simulink model "SVPWM"  (R2021a)
settings: Solver=FixedStepAuto  StartTime=0.0  StopTime=0.02  FixedStep=1e-7  RelTol=1e-3
values from neighbouring files (symbols this model uses):
  f_fund = 50    [run_sim.m]
  ma = 0.2    [run_sim.m]
  phaseA = 0    [run_sim.m]
  phi_carrier = 0    [run_sim.m]
libraries: dspxfrm3 x1, mcbcontrolslib x1, spsTriangleGeneratorLib x1, spsabctoAlphaBetaZeroLib x1
settings Model: Creator=enes_  LastModifiedBy=enes_

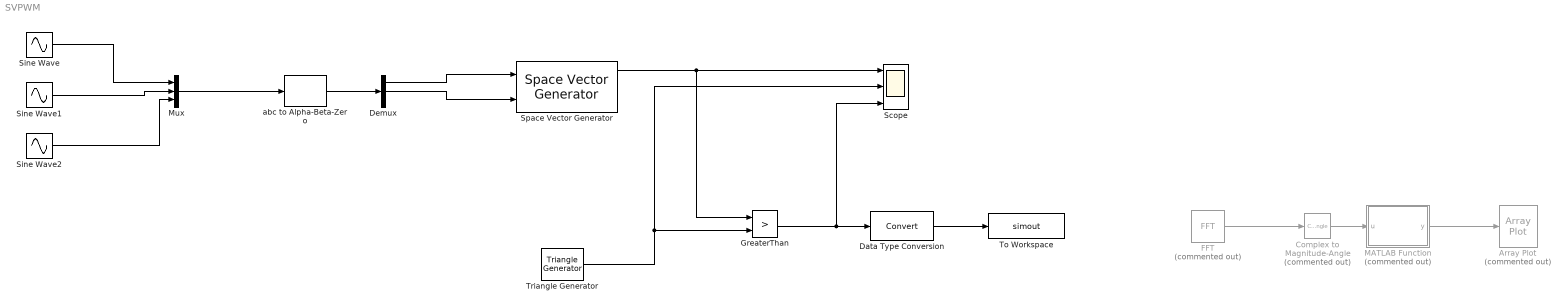
== system SVPWM ==
  Array Plot : ArrayPlot  Commented=on  WindowPosition=[503.000000,290.000000,800.000000,500.000000,]  DefaultConfigurationName=dsp.scopes.ArrayPlotBlockSpecification
  Complex to Magnitude-Angle : ComplexToMagnitudeAngle  Commented=on  Output=Magnitude
  Data Type Conversion : DataTypeConversion
  Demux : Demux  Outputs=3
  FFT : dspxfrm3/FFT  Commented=on  FFTImplementation=Auto  CompMethod=Table lookup  TableOpt=NEW  TableOptActive=Speed  BitRevOrder=off  Normalize=off  InheritFFTLength=on  FFTLength=64  WrapInput=on  roundingMode=Floor  overflowMode=off  firstCoeffDataTypeStr=Inherit: Same word length as input  firstCoeffLastDataTypeStr=Inherit: Same word length as input  outputMin=[]  outputMax=[]
  GreaterThan : RelationalOperator  Operator=>  OutDataTypeStr=boolean  RndMeth=Simplest
  MATLAB Function : MATLAB Function  Commented=on  TreatAsAtomicUnit=on
  Mux : Mux  Inputs=3
  Scope : Scope  NumInputPorts=3
  Sine Wave : Sin  Amplitude=ma  Frequency=2*pi*f_fund  Phase=phaseA  SampleTime=0
  Sine Wave1 : Sin  Amplitude=ma  Frequency=2*pi*f_fund  Phase=-2*pi/3+phaseA  SampleTime=0
  Sine Wave2 : Sin  Amplitude=ma  Frequency=2*pi*f_fund  Phase=2*pi/3+phaseA  SampleTime=0
  Space Vector Generator : mcbcontrolslib/Space Vector Generator
      settings: SourceProductBaseCode=MT
  To Workspace : ToWorkspace  VariableName=simout  SaveFormat=Timeseries  SampleTime=-1
  Triangle Generator : spsTriangleGeneratorLib/Triangle Generator  Freq=f_carrier  Phase=90+phi_carrier  Ts=0
  abc to Alpha-Beta-Zero : spsabctoAlphaBetaZeroLib/abc to Alpha-Beta-Zero
      settings: SourceProductBaseCode=PS
  wires:
  Sine Wave/1 -> Mux/1
  Sine Wave1/1 -> Mux/2
  Sine Wave2/1 -> Mux/3
  Mux/1 -> abc to Alpha-Beta-Zero/1
  abc to Alpha-Beta-Zero/1 -> Demux/1
  Demux/1 -> Space Vector Generator/1
  Demux/2 -> Space Vector Generator/2
  Space Vector Generator/1 -> GreaterThan/1, Scope/1
  Triangle Generator/1 -> GreaterThan/2, Scope/2
  GreaterThan/1 -> Data Type Conversion/1, Scope/3
  FFT/1 -> Complex to Magnitude-Angle/1
  Complex to Magnitude-Angle/1 -> MATLAB Function/1(u)
  MATLAB Function/1(y) -> Array Plot/1
  Data Type Conversion/1 -> To Workspace/1

== matlab function SVPWM/MATLAB Function ==
  data: u input; y output
function y = fcn(u)

y = fftshift(u);
